simulink model "RobotModel5"  (R2025b)
settings: Solver=VariableStepAuto  StartTime=0.0  StopTime=40  RelTol=0.01  AbsTol=0.01  EnableMultiTasking=on
values from neighbouring files (symbols this model uses):
  waypoints = [R*cos(theta)+5, R*sin(theta)]    [init_waypoints.m]
undefined symbols (not defined in the file or in its folder): X, Y, Z
libraries: sm_lib x58, nesl_utility x45, slpidlib x2, robotalgslib x1, sharedtransform x1
(part 4 of 4)

== matlab function RobotModel5/Subsystem2/MATLAB Function1 ==
  data: mode_cmd input; alpha input; tau output; q input; dq input; q_cmd input; is_locked output; q_ref output
function [tau, is_locked, q_ref] = LockJointPD(mode_cmd, alpha, q, dq, q_cmd)
%#codegen
% mode_cmd: 0=Walk (track q_cmd), 1=Wheeled (lock current angle)
% alpha   : [0,1] smoothing factor (TransferFcn output), 0=fully walking, 1=fully locked
% q,dq    : joint angle/angular velocity
% q_cmd   : walk/stand target angle (radians)
Kp = 1200.0;   % Starting value, tune per joint
Kd =   20.0;
tau_lim = 300.0;
m = uint8(mode_cmd ~= 0);     % Standardize to uint8(0/1)
a = double(alpha);
persistent q_hold last_mode
if isempty(q_hold),    q_hold    = q;        end   % double
if isempty(last_mode), last_mode = uint8(0); end   % uint8
% Rising edge: 0->1, latch current angle
if (last_mode == uint8(0)) && (m ~= uint8(0))
    q_hold = q;
end
last_mode = m;
% Reference angle: interpolate between "hold angle" and "target angle"
q_ref  = a*q_hold + (1-a)*q_cmd;
dq_ref = 0.0;
% PD
tau = Kp*(q_ref - q) + Kd*(dq_ref - dq);
% Saturation
tau = max(min(tau, tau_lim), -tau_lim);
% Debug flag: is leg lock dominant
is_locked = (a > 0.5);     % Can also output m==1
end

== matlab function RobotModel5/Subsystem3/MATLAB Function ==
  data: mode_cmd input; alpha input; tau output; q input; dq input; q_cmd input; is_locked output; q_ref output
function [tau, is_locked, q_ref] = LockJointPD(mode_cmd, alpha, q, dq, q_cmd)
%#codegen
% mode_cmd: 0=Walk (track q_cmd), 1=Wheeled (lock current angle)
% alpha   : [0,1] smoothing factor (TransferFcn output), 0=fully walking, 1=fully locked
% q,dq    : joint angle/angular velocity
% q_cmd   : walk/stand target angle (radians)
Kp = 1200.0;   % Starting value, tune per joint
Kd =   20.0;
tau_lim = 300.0;
m = uint8(mode_cmd ~= 0);     % Standardize to uint8(0/1)
a = double(alpha);
persistent q_hold last_mode
if isempty(q_hold),    q_hold    = q;        end   % double
if isempty(last_mode), last_mode = uint8(0); end   % uint8
% Rising edge: 0->1, latch current angle
if (last_mode == uint8(0)) && (m ~= uint8(0))
    q_hold = q;
end
last_mode = m;
% Reference angle: interpolate between "hold angle" and "target angle"
q_ref  = a*q_hold + (1-a)*q_cmd;
dq_ref = 0.0;
% PD
tau = Kp*(q_ref - q) + Kd*(dq_ref - dq);
% Saturation
tau = max(min(tau, tau_lim), -tau_lim);
% Debug flag: is leg lock dominant
is_locked = (a > 0.5);     % Can also output m==1
end

== matlab function RobotModel5/Subsystem3/MATLAB Function1 ==
  data: mode_cmd input; alpha input; tau output; q input; dq input; q_cmd input; is_locked output; q_ref output
function [tau, is_locked, q_ref] = LockJointPD(mode_cmd, alpha, q, dq, q_cmd)
%#codegen
% mode_cmd: 0=Walk (track q_cmd), 1=Wheeled (lock current angle)
% alpha   : [0,1] smoothing factor (TransferFcn output), 0=fully walking, 1=fully locked
% q,dq    : joint angle/angular velocity
% q_cmd   : walk/stand target angle (radians)
Kp = 1200.0;   % Starting value, tune per joint
Kd =   20.0;
tau_lim = 300.0;
m = uint8(mode_cmd ~= 0);     % Standardize to uint8(0/1)
a = double(alpha);
persistent q_hold last_mode
if isempty(q_hold),    q_hold    = q;        end   % double
if isempty(last_mode), last_mode = uint8(0); end   % uint8
% Rising edge: 0->1, latch current angle
if (last_mode == uint8(0)) && (m ~= uint8(0))
    q_hold = q;
end
last_mode = m;
% Reference angle: interpolate between "hold angle" and "target angle"
q_ref  = a*q_hold + (1-a)*q_cmd;
dq_ref = 0.0;
% PD
tau = Kp*(q_ref - q) + Kd*(dq_ref - dq);
% Saturation
tau = max(min(tau, tau_lim), -tau_lim);
% Debug flag: is leg lock dominant
is_locked = (a > 0.5);     % Can also output m==1
end

== matlab function RobotModel5/Subsystem4/MATLAB Function ==
  data: mode_cmd input; alpha input; tau output; q input; dq input; q_cmd input; is_locked output; q_ref output
function [tau, is_locked, q_ref] = LockJointPD(mode_cmd, alpha, q, dq, q_cmd)
%#codegen
% mode_cmd: 0=Walk (track q_cmd), 1=Wheeled (lock current angle)
% alpha   : [0,1] smoothing factor (TransferFcn output), 0=fully walking, 1=fully locked
% q,dq    : joint angle/angular velocity
% q_cmd   : walk/stand target angle (radians)
Kp = 1200.0;   % Starting value, tune per joint
Kd =   20.0;
tau_lim = 300.0;
m = uint8(mode_cmd ~= 0);     % Standardize to uint8(0/1)
a = double(alpha);
persistent q_hold last_mode
if isempty(q_hold),    q_hold    = q;        end   % double
if isempty(last_mode), last_mode = uint8(0); end   % uint8
% Rising edge: 0->1, latch current angle
if (last_mode == uint8(0)) && (m ~= uint8(0))
    q_hold = q;
end
last_mode = m;
% Reference angle: interpolate between "hold angle" and "target angle"
q_ref  = a*q_hold + (1-a)*q_cmd;
dq_ref = 0.0;
% PD
tau = Kp*(q_ref - q) + Kd*(dq_ref - dq);
% Saturation
tau = max(min(tau, tau_lim), -tau_lim);
% Debug flag: is leg lock dominant
is_locked = (a > 0.5);     % Can also output m==1
end
